simulink model "followerStopper"  (R2018b)
settings: Solver=FixedStepAuto  StartTime=0.0  StopTime=inf  FixedStep=0.05  RelTol=1e-3  EnableMultiTasking=on
undefined symbols (not defined in the file or in its folder): Angular, Linear
libraries: robotlib x8
settings Model: Creator=sprinkle  LastModifiedBy=ckreienk
settings OptimizationCC: LifeSpan=Inf  MaxStackSize=64
settings DebuggingCC: LibraryContextMissingDiagnostic=none  SFUnexpectedBacktrackingDiag=warning  SFNoUnconditionalDefaultTransitionDiag=warning  SFExecutionAtInitializationDiag=none
settings HardwareCC: ProdBitPerPointer=32  ProdBitPerSizeT=32  ProdBitPerPtrDiffT=32  ProdLargestAtomicFloat=None  ProdIntDivRoundTo=Undefined  ProdEndianess=Unspecified  ProdWordSize=32  ProdHWDeviceType=Generic->Unspecified (assume 32-bit Generic)
settings SFSimCC: SimUseLocalCustomCode=off  MATLABDynamicMemAlloc=off
settings RTWCC: SystemTargetFile=ert.tlc  HardwareBoard=Robot Operating System (ROS)  TLCOptions=-aInlineSetEventsForThisBaseRateFcn=TLC_FALSE -aSuppressMultiTaskScheduler=TLC_FALSE -aRateBasedStepFcn=0  TemplateMakefile=ert_default_tmf  GenerateReport=on  RTWUseLocalCustomCode=off  Toolchain=Catkin  IncludeHyperlinkInReport=on  LaunchReport=on  TargetLang=C++  GenerateTraceInfo=on  GenerateTraceReport=on  GenerateTraceReportSl=on  GenerateTraceReportSf=on  GenerateTraceReportEml=on
settings CodeAppCC: ForceParamTrailComments=on  IgnoreCustomStorageClasses=off  OperatorAnnotations=on  SimulinkDataObjDesc=on  SFDataObjDesc=on  MATLABFcnDesc=on  InsertBlockDesc=on  StateflowObjectComments=on  MATLABSourceComments=on
settings ERTTargetCC: MultiwordLength=2048
settings ConfigComp: CovMetricSettings=dw  CovHtmlReporting=on  CovSaveCumulativeToWorkspaceVar=on  CovSaveSingleToWorkspaceVar=on  CovExternalEMLEnable=off

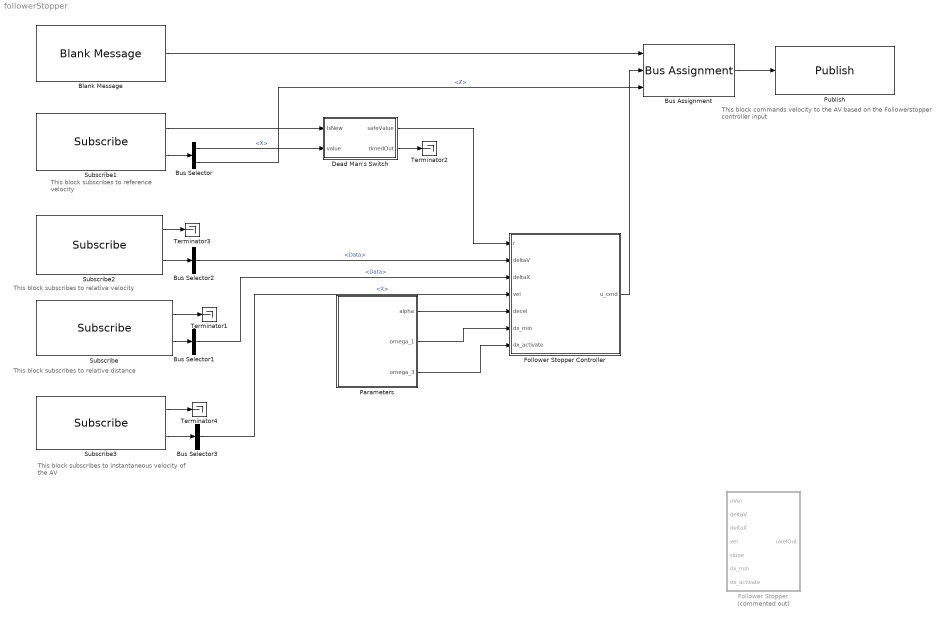
== system followerStopper ==
  note: This block subscribes
      | to reference velocity
  note: This block subscribes to relative velocity
  note: This block subscribes to relative distance
  note: This block subscribes to
      | instantaneous velocity of the AV
  note: This block commands velocity to the AV based
      | on the Followerstopper controller input
  Blank Message : robotlib/Blank Message  messageClass=Message  entityType=geometry_msgs/Twist  messageType=geometry_msgs/Twist  SampleTime=inf
      settings: SourceProductBaseCode=RO
  Bus Assignment : BusAssignment  AssignedSignals=Linear.X,Angular.Z
  Bus Selector : BusSelector  OutputSignals=Linear.X,Angular.Z
  Bus Selector1 : BusSelector  OutputSignals=Data
  Bus Selector2 : BusSelector  OutputSignals=Data
  Bus Selector3 : BusSelector  OutputSignals=Linear.X
  Dead Man's Switch : Subsystem  TreatAsAtomicUnit=on  mask{stepSize=0.05, timeout=0.2}
      mask prompts: stepSize "Simulation step size"; timeout "Timeout (in seconds)"
      mask help: Interprets whether a new message has been recently received, and if so permits the data in 'value' to be passed through. Otherwise, 0 is outputted from 'safeValue'
      mask Help: Interprets whether a new message has been recently received, and if so permits the data in 'value' to be passed through. Otherwise, 0 is outputted from 'safeValue'
  Follower Stopper : Subsystem  Commented=on
  Follower Stopper Controller : Subsystem
  Parameters : Subsystem
  Publish : robotlib/Publish  topicSource=Specify your own  topic=cmd_vel_wrench  messageType=geometry_msgs/Twist  messageQueueLength=1
      settings: SourceProductBaseCode=RO
  Subscribe : robotlib/Subscribe  topicSource=Specify your own  topic=kalmanFilter/dist  messageType=std_msgs/Float32  sampleTime=-1  messageQueueLength=1
      settings: SourceProductBaseCode=RO
  Subscribe1 : robotlib/Subscribe  topicSource=Specify your own  topic=cmd_vel_wrench_in  messageType=geometry_msgs/Twist  sampleTime=-1  messageQueueLength=1
      settings: SourceProductBaseCode=RO
  Subscribe2 : robotlib/Subscribe  topicSource=Specify your own  topic=kalmanFilter/vel  messageType=std_msgs/Float32  sampleTime=-1  messageQueueLength=1
      settings: SourceProductBaseCode=RO
  Subscribe3 : robotlib/Subscribe  topicSource=Specify your own  topic=vel  messageType=geometry_msgs/Twist  sampleTime=-1  messageQueueLength=1
      settings: SourceProductBaseCode=RO
  Terminator{1..4} (4 alike) : Terminator
  wires:
  Subscribe1/2 -> Bus Selector/1
  Subscribe1/1 -> Dead Man's Switch/1(IsNew)
  Blank Message/1 -> Bus Assignment/1
  Bus Assignment/1 -> Publish/1
  Follower Stopper Controller/1(u_cmd) -> Bus Assignment/2
  Subscribe/1 -> Terminator1/1
  Subscribe/2 -> Bus Selector1/1
  Dead Man's Switch/1(safeValue) -> Follower Stopper Controller/1(r)
  Bus Selector/1 -> Dead Man's Switch/2(value)  "<X>"
  Dead Man's Switch/2(timedOut) -> Terminator2/1
  Subscribe2/1 -> Terminator3/1
  Subscribe2/2 -> Bus Selector2/1
  Subscribe3/1 -> Terminator4/1
  Subscribe3/2 -> Bus Selector3/1
  Bus Selector2/1 -> Follower Stopper Controller/2(deltaV)  "<Data>"
  Bus Selector1/1 -> Follower Stopper Controller/3(deltaX)  "<Data>"
  Bus Selector3/1 -> Follower Stopper Controller/4(vel)  "<X>"
  Bus Selector/2 -> Bus Assignment/3  "<Z>"
  Parameters/1(alpha) -> Follower Stopper Controller/5(decel)
  Parameters/2(omega_1) -> Follower Stopper Controller/6(dx_min)
  Parameters/3(omega_3) -> Follower Stopper Controller/7(dx_activate)

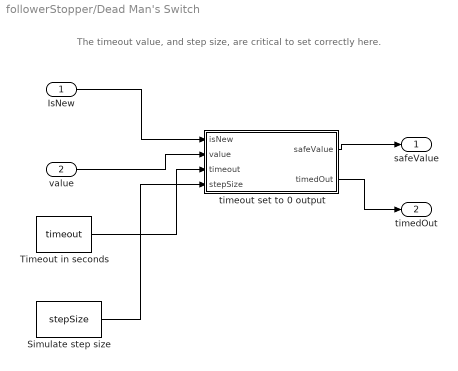
== system followerStopper/Dead Man's Switch ==
  note: The timeout value, and step size, are critical to set correctly here.
  IsNew : Inport
  value : Inport  Port=2
  Simulate step size : Constant  Value=stepSize
  Timeout in seconds : Constant  Value=timeout
  timeout set to 0 output : MATLAB Function  TreatAsAtomicUnit=on
  safeValue : Outport  InitialOutput=[0]
  timedOut : Outport  Port=2  InitialOutput=[0]
  wires:
  IsNew/1 -> timeout set to 0 output/1(isNew)
  timeout set to 0 output/1(safeValue) -> safeValue/1
  value/1 -> timeout set to 0 output/2(value)
  Timeout in seconds/1 -> timeout set to 0 output/3(timeout)
  timeout set to 0 output/2(timedOut) -> timedOut/1
  Simulate step size/1 -> timeout set to 0 output/4(stepSize)

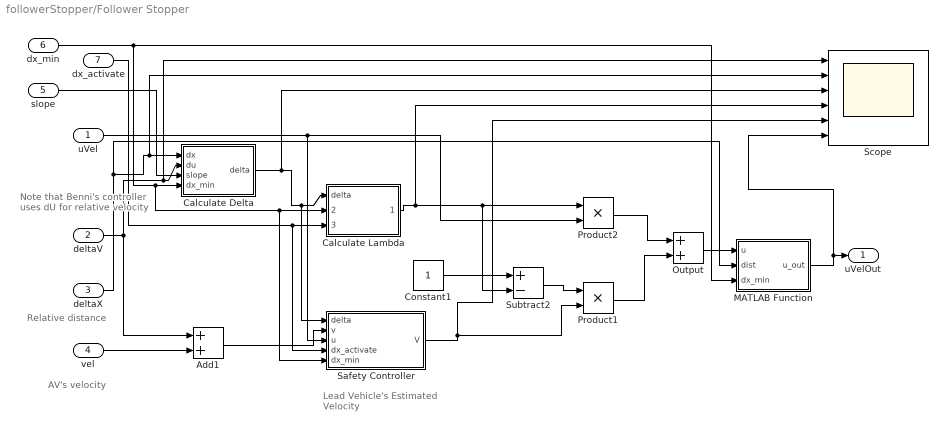
== system followerStopper/Follower Stopper ==
  note: Relative distance
  note: AV's velocity
  note: Lead Vehicle's
      | Estimated Velocity
  note: Note that Benni's
      | controller uses dU
      | for relative
      | velocity
  uVel : Inport
  deltaV : Inport  Port=2
  deltaX : Inport  Port=3
  vel : Inport  Port=4
  slope : Inport  Port=5
  dx_min : Inport  Port=6
  dx_activate : Inport  Port=7
  Add1 : Sum
  Calculate Delta : MATLAB Function  TreatAsAtomicUnit=on
  Calculate Lambda : MATLAB Function  TreatAsAtomicUnit=on
  Constant1 : Constant  SampleTime=-1
  MATLAB Function : MATLAB Function  TreatAsAtomicUnit=on
  Output : Sum
  Product1 : Product
  Product2 : Product
  Safety Controller : MATLAB Function  TreatAsAtomicUnit=on
  Scope : Scope  NumInputPorts=6
  Subtract2 : Sum  Inputs=+-
  uVelOut : Outport
  wires:
  deltaX/1 -> MATLAB Function/2(dist), Scope/2, Calculate Delta/1(dx)
  deltaV/1 -> Add1/1, Scope/1, Calculate Delta/2(du)
  Calculate Delta/1(delta) -> Scope/3, Safety Controller/1(delta), Calculate Lambda/1(delta)
  Add1/1 -> Safety Controller/2(v)
  Safety Controller/1(V) -> Scope/5, Product1/2
  Calculate Lambda/1(lambda) -> Scope/4, Subtract2/2, Product2/1
  Constant1/1 -> Subtract2/1
  Subtract2/1 -> Product1/1
  uVel/1 -> Safety Controller/3(u), Product2/2
  Product2/1 -> Output/1
  Product1/1 -> Output/2
  Output/1 -> MATLAB Function/1(u)
  vel/1 -> Add1/2
  dx_min/1 -> MATLAB Function/3(dx_min), Safety Controller/5(dx_min), Calculate Lambda/2(dx_min), Calculate Delta/4(dx_min)
  slope/1 -> Calculate Delta/3(slope)
  dx_activate/1 -> Safety Controller/4(dx_activate), Calculate Lambda/3(dx_activate)
  MATLAB Function/1(u_out) -> Scope/6, uVelOut/1

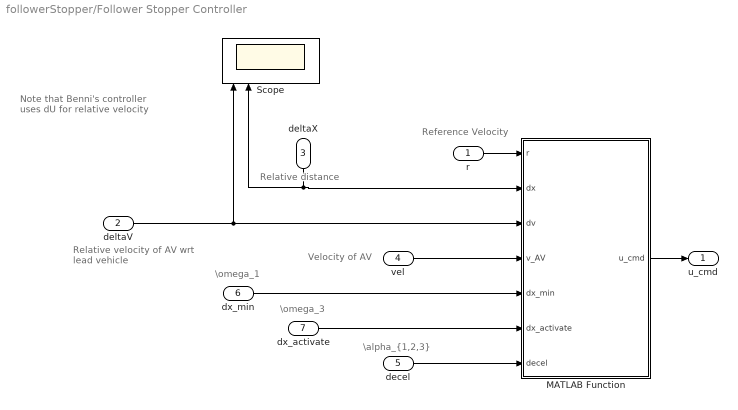
== system followerStopper/Follower Stopper Controller ==
  note: Note that Benni's
      | controller uses dU
      | for relative
      | velocity
  note: Relative velocity of
      | AV wrt lead vehicle
  note: Velocity of AV
  note: Reference Velocity
  note: Relative distance
  note: \omega_1
  note: \omega_3
  note: \alpha_{1,2,3}
  r : Inport
  deltaV : Inport  Port=2
  deltaX : Inport  Port=3
  vel : Inport  Port=4
  decel : Inport  Port=5
  dx_min : Inport  Port=6
  dx_activate : Inport  Port=7
  MATLAB Function : MATLAB Function  TreatAsAtomicUnit=on
  Scope : Scope  NumInputPorts=6
  u_cmd : Outport
  wires:
  deltaX/1 -> MATLAB Function/2(dx), Scope/2
  deltaV/1 -> MATLAB Function/3(dv), Scope/1
  MATLAB Function/1(u_cmd) -> u_cmd/1
  vel/1 -> MATLAB Function/4(v_AV)
  dx_min/1 -> MATLAB Function/5(dx_min)
  decel/1 -> MATLAB Function/7(decel)
  dx_activate/1 -> MATLAB Function/6(dx_activate)
  r/1 -> MATLAB Function/1(r)

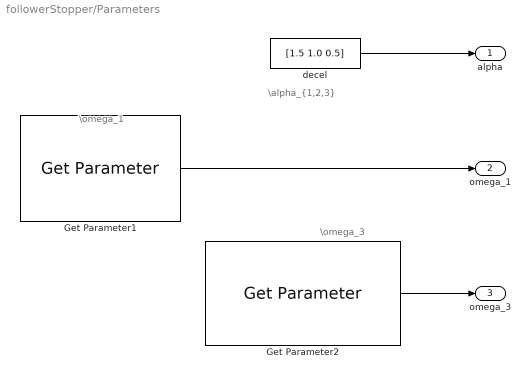
== system followerStopper/Parameters ==
  note: \omega_3
  note: \omega_1
  note: \alpha_{1,2,3}
  Get Parameter1 : robotlib/Get Parameter  ParameterSource=Specify your own  ParameterName=/dx_min  ParameterType=double  ParameterMaxArrayLength=16  ParameterInitialValue=4.5  SampleTime=-1  ShowErrorCodeOutput=off  ModelName=followerStopper  BlockId=ParamGet_followerStopper_129
      settings: SourceProductName=Robotics System Toolbox  SourceProductBaseCode=RO
  Get Parameter2 : robotlib/Get Parameter  ParameterSource=Specify your own  ParameterName=/dx_activate  ParameterType=double  ParameterMaxArrayLength=16  ParameterInitialValue=6.0  SampleTime=-1  ShowErrorCodeOutput=off  ModelName=followerStopper  BlockId=ParamGet_followerStopper_130
      settings: SourceProductName=Robotics System Toolbox  SourceProductBaseCode=RO
  decel : Constant  Value=[1.5 1.0 0.5]  OutDataTypeStr=double  SampleTime=-1
  alpha : Outport
  omega_1 : Outport  Port=2
  omega_3 : Outport  Port=3
  wires:
  Get Parameter2/1 -> omega_3/1
  Get Parameter1/1 -> omega_1/1
  decel/1 -> alpha/1

== matlab function followerStopper/Follower Stopper/Calculate Lambda ==
  data: delta input; lambda output; dx_min input; dx_activate input
function lambda = fcn(delta,dx_min,dx_activate)
%#codegen
dx_mid = (dx_activate+dx_min)/2;
% Based on a controller by Benni Seibold
% MATLAB by Jonathan Sprinkle

lambda = min(max((delta-dx_min)/(dx_activate-dx_min),0),1);
assert(lambda<=1);
% to see this plotted:
% 
% delta=linspace(0,25);
% lambda = min(max(delta/2 - 1.5,0),1);
% figure
% plot(delta,lambda)
% axis([-0.5 20 -1 3])
% title('\lambda as a function of \Delta')

== matlab function followerStopper/Dead Man's Switch/timeout set to 0 output ==
  data: isNew input; safeValue output; value input; timeout input; timedOut output; stepSize input
function [safeValue,timedOut] = fcn(isNew,value,timeout,stepSize)
%#codegen
persistent sinceLastMsg
timedOut=true;
if isempty(sinceLastMsg)
    sinceLastMsg=(timeout/stepSize)+1;
end

safeValue=0;
% if no new message
% after timeout, we output 0
if( isNew == true )
    sinceLastMsg = 0;
else
    sinceLastMsg = sinceLastMsg+1;
end

% Note: we require step size as an input here, and depend on our
% system being executed at a regular rate, or bad things will happen
if( sinceLastMsg < timeout/stepSize )
    timedOut = false;
end
    
if( timedOut == false )
    safeValue = value;
end

== matlab function followerStopper/Follower Stopper/Safety Controller ==
  data: delta input; V output; v input; u input; dx_activate input; dx_min input
function V = fcn(delta,v,u,dx_activate,dx_min)
%#codegen
dx_mid = (dx_activate+dx_min)/2;

V = v*min(max((delta-dx_min)/(dx_mid-dx_min),0),1);
V = min(V,u);

== matlab function followerStopper/Follower Stopper/Calculate Delta ==
  data: dx input; delta output; du input; slope input; dx_min input
function delta = fcn(dx,du,slope,dx_min)
%#codegen

% Based on a controller by Benni Seibold
% MATLAB by Jonathan Sprinkle

delta = dx + (slope)*du;
% delta = dx - (4/3)*du;

if( dx < dx_min )
    delta = single(1);
end

% to see this plotted:
% 
% [du,dx] = meshgrid(-8:0.1:8,0:0.1:5);
% delta = dx - (4/3)*du;
% figure
% surf(du,dx,delta)
% xlabel('du')
% ylabel('dx')
% zlabel('\Delta')

== matlab function followerStopper/Follower Stopper/MATLAB Function ==
  data: u input; u_out output; dist input; dx_min input
function u_out = fcn(u,dist,dx_min)
%#codegen
if( dist <= dx_min )
    u_out = 0;
else
    u_out = u;
end

== matlab function followerStopper/Follower Stopper Controller/MATLAB Function ==
  data: r input; u_cmd output; dx input; dv input; v_AV input; dx_min input; dx_activate input; decel input
function u_cmd = fcn(r,dx,dv,v_AV,...
    dx_min,dx_activate,decel)
%#codegen
% Safety controller, based on quadratic bands.
% Input: r = desired velocity (from other models)
%          dx = estimate of gap to vehicle ahead
%          dv = estimate of time derivative of dx (= velocity difference)
%         v_AV = velocity of AV
%      dx_min = minimum distance
% dx_activate = distance below which controller does something
%       decel = vector of three deceleration values for parabolas
% Out:  u_cmd = actual velocity commanded (always u_cmd<=U)
%
% Controller-specific parameters
dx_mid = (dx_min+dx_activate)/2; % mid distance, where v_lead is commanded
% Lead vehicle velocity
v_lead = v_AV+dv; % velocity of lead vehicle
v_lead = max(v_lead,0); % lead vehicle cannot go backwards
v = min(r,v_lead); % safety velocity cannot exceed desired velocity U
% Treatment of positive dv-values
dv = min(dv,0); % domains for dv>0 same as dv=0
% For given dv, dx-values of band boundaries
dx1 = dx_min+1/(2*decel(1))*dv.^2;
dx2 = dx_mid+1/(2*decel(2))*dv.^2;
dx3 = dx_activate+1/(2*decel(3))*dv.^2;
% Actual commanded velocity
u_cmd = double((dx1<dx&dx<=dx2).*(v.*(dx-dx1)./(dx2-dx1))+...
    (dx2<dx&dx<=dx3).*(v+(r-v).*(dx-dx2)./(dx3-dx2))+...
    (dx3<dx).*r);
% DO not move if within dx_min
% if(dx < dx_min)
%     u_cmd = 0;
% end

if( dx > 16.0 )
    u_cmd = r;
end
